simulink model "Milford"  (R2017a)
settings: Solver=FixedStepAuto  StartTime=0.0  StopTime=Cycle_End  FixedStep=0.01  MaxStep=0.01  RelTol=1e-3  EnableMultiTasking=on
PostLoadFcn:
  | , if any(exist('dsrtsu_mdlpostloadfcn', 'file') == [2, 3, 6]), try dsrtsu_mdlpostloadfcn('Execute', bdroot); catch fprintf('Error in PostLoadFcn (dsrtsu_mdlpostloadfcn) for model "%s":\n %s\n', bdroot, lasterr); end, end,
undefined symbols (not defined in the file): Actuators, APP1_OOR, APP2_OOR, APP_Mismatch, Brk_Flt, cal, ClutchEngag, DiscIntNeverNeededParam, eng, Engine, EngOverTemp, ENGTRQ_MSMCH_Degraded_CP, ENGTRQ_MSMCH_ErrCritical_CP, ENGTRQ_MSMCH_LimpHome_CP, EngTrqMismatch, ESSOverTemp, gb, Gearbox, KeyPos_Flt, lib_Actuators, lib_Sensors_2017a, lib_Transmission, Loss, LossCAN, MCUOverTemp, mot, MotDirMismatch, MotOverTemp, MotTrqMismatch, mph2kph, PRNDL_Flt, Ratio, RegenFault, Sensors, Spd, time, Transmission
libraries: simulink x110, powerlib_meascontrol x6, EC2_libraries x5, dspsigops x3, lib_Chassis x1, lib_DCDC x1, lib_Differential x1, lib_HVESS x1, lib_Engine x1, lib_OBC x1, Transmission_Validation x1, lib_Wheels x1
(part 9 of 9)

== stateflow chart Milford/Controller_with_Transmission_Manager1/HSC/Powertrain Manager/HV Manager/BMS_Manager/ESS_Manager ==
  state Fault_light_OFF
    entry: GFD_Light=0;
  state Ground_Fault
    entry:
    HV_State=-7;
    GFD_Light=1
  state Voltage_Fault
  state HVIL_Fault
    entry: MO_BMS_Sollmodus=0;
    HV_State=-8
  state HV_Startup
    state Drive_State
      entry:  HV_State=1;
      T_15=1;
      T_30=1;
      HVDischarge=0;
    state Contactor
      entry:
      T_30C=1;
    state Clear_Faults
      entry:
      Diag_Rq_Fktnl_Data_OBD_byte_0 =1;
      Diag_Rq_Fktnl_Data_OBD_byte_1=4;
      Diag_Rq_Fktnl_Data_OBD_byte_2=0;
      Diag_Rq_Fktnl_Data_OBD_byte_3=0;
      Diag_Rq_Fktnl_Data_OBD_byte_4=0;
      Diag_Rq_Fktnl_Data_OBD_byte_5=0;
      Diag_Rq_Fktnl_Data_OBD_byte_6=0;
      Diag_Rq_Fktnl_Data_OBD_byte_7=0;
      HV_State=2;
    state Charge_Wake
      entry: chga_wake=1;
      HV_State=3;
    state Drive_Wake
      entry: veh_wake=1;
      HV_State=8;
    state BMS_Enable_Charge
      entry: MO_BMS_Sollmodus=0;
      % T_15=1;
      % T_30C=1;
      HV_State=4;
    state BMS_Enable_Drive
      entry: MO_BMS_Sollmodus=0;
      HV_State=9;
    state Power_Contactors_Drive
      en: MO_BMS_Sollmodus=0;
      HV_State=10;
    state Power_Contactors_Charge
      en: MO_BMS_Sollmodus=0;
      %T_30C=1;
      HV_State=5;
    state Close_Contactors_Drive
      entry:
      MO_BMS_Sollmodus=1;
      HV_State=11;
    state Close_Contactors_Charge
      entry:
      MO_BMS_Sollmodus=1;
      HV_State=6;
    state Time_delay
    state Ready_to_Charge
      entry: ReadyToCharge=1;
      ISO_Hybrid_01_Req = 1;
      HV_State=7;
    state Ready_to_Drive
      entry: ReadyToDrive=1;
      ISO_Hybrid_01_Req = 1;
      HV_State=12;
    (default) -> Contactor
    Contactor -> Drive_State : after(0.25,sec)
    Drive_State -> Clear_Faults : after(0.1,sec)
    Clear_Faults -> Charge_Wake [order 1] : [plugged]
    Clear_Faults -> Drive_Wake [order 2] : %after(0.1,sec)
    Drive_Wake -> BMS_Enable_Drive : [BMS_Fehler_Pilot==0 ]
    Charge_Wake -> BMS_Enable_Charge : [BMS_Fehler_Pilot==0 ]
    BMS_Enable_Charge -> Power_Contactors_Charge : [BMS_Init_abgeschlossen]
    BMS_Enable_Drive -> Power_Contactors_Drive : [BMS_Init_abgeschlossen]
    Power_Contactors_Drive -> Close_Contactors_Drive : [closeMaincReq]
    Power_Contactors_Charge -> Close_Contactors_Charge : [closeMaincReq]
    Close_Contactors_Charge -> Time_delay : [BMS_Fehler_HS_offen==0&&(BMS_IstModus==4||BMS_IstModus==1)]
    Close_Contactors_Drive -> Ready_to_Drive : [BMS_Fehler_HS_offen==0&&BMS_IstModus==1]
    Time_delay -> Ready_to_Charge : after(1,sec)
    Ready_to_Drive -> Ready_to_Charge : [plugged]
    Ready_to_Charge -> Ready_to_Drive : [plugged==0]
  note: // Rev 2_14_2017
      | Added plugged to Off-On transition
      | Added EnableInverter to charge path
      | Changed IstModus to 1 at the end of charge path
      |
      | Create HV On Request block to request charging when vehicle is off
  state HV_Shudown
    state Open_Contactors
      entry: MO_BMS_Sollmodus=0;
      HV_State=-1;
      ISO_Hybrid_01_Req = 0;
    state ShutDown_T30C
      entry: T_30C=0;
    state Discharge_Bus
      entry: HVDischarge=1;
      HV_State=-2;
    state Disable_BCM_1
      entry: T_15=0;
      HVDischarge=0;
      HV_State=-3;
    state Disable_BCM_2
      entry: T_30=0;
      HVDischarge=0;
      HV_State=-4;
    state Send_BCM_to_Sleep
      en: MO_SleepAckn =1;
      T_15=0;
      T_30=0;
      HV_State=-5;
    state Shutdown_Complete
      entry: Shutdown_Complete=1;
      HV_State=-6;
    (default) -> Open_Contactors
    Open_Contactors -> ShutDown_T30C : after(2,sec)
    ShutDown_T30C -> Discharge_Bus : [BMS_IstModus==5]
    Discharge_Bus -> Disable_BCM_1 : [BMS_Spannung_ZwKr<30]
    Disable_BCM_1 -> Disable_BCM_2 : [BMS_IstStrom<0.02]
    Disable_BCM_2 -> Send_BCM_to_Sleep
    Send_BCM_to_Sleep -> Shutdown_Complete : [BMS_SleepInd]
  note: //Rev 8_21_2017
      | //Removed all engine related conditions
      | //Removed EngRunATV
  Voltage_Fault -> HV_Shudown [order 1] : after(0.5, sec)
  Ground_Fault -> Fault_light_OFF : [(ISOfault==0&&KeyPos==1)||(ISOfault==0&&KeyPos==0&&plugged==1)]
  HV_Shudown -> Ground_Fault [order 2] : [ISOfault==1]
  Fault_light_OFF -> HV_Shudown
  HV_Startup -> Ground_Fault [order 3] : [ISOfault==1]
  HV_Startup -> HVIL_Fault [order 4] : [BMS_Fehler_Pilot]
  HVIL_Fault -> HV_Shudown : [BMS_Fehler_Pilot==0]
  HV_Startup -> Voltage_Fault [order 2] : after(5,sec)
      | [BMS_Spannung_ZwKr<50&&EngRunAtv]
  Voltage_Fault -> HV_Startup [order 2] : after(1,sec)
  (default) -> HV_Shudown
  HV_Shudown -> HV_Startup [order 1] : [HV_req==1||plugged||EngRunAtv]
  HV_Startup -> HV_Shudown [order 1] : [closeMaincReq==0&&plugged==0]
      | {ReadyToDrive = 0;
      | ReadyToCharge = 0;}
  data: data local; ISOfault input; plugged input; BMS_Fehler_HS_offen input; BMS_Fehler_Pilot input; BMS_Init_abgeschlossen input; BMS_IstModus input; BMS_IstSpannung input; BMS_IstStrom input; BMS_SleepInd input; Diag_Rq_Fktnl_Data_OBD_byte_0 output; Diag_Rq_Fktnl_Data_OBD_byte_1 output; Diag_Rq_Fktnl_Data_OBD_byte_2 output; Diag_Rq_Fktnl_Data_OBD_byte_3 output; Diag_Rq_Fktnl_Data_OBD_byte_4 output; Diag_Rq_Fktnl_Data_OBD_byte_5 output; Diag_Rq_Fktnl_Data_OBD_byte_6 output; Diag_Rq_Fktnl_Data_OBD_byte_7 output; ISO_Hybrid_01_Req output; MO_SleepAckn output; MO_BMS_Sollmodus output; T_15 output; T_30 output; T_30C output; veh_wake output; chga_wake output; HVDischarge output; HV_State output; ReadyToDrive output; ReadyToCharge output; Shutdown_Complete output; HV_req input boolean; BMS_Spannung_ZwKr input; NMH_BMS_Car_WakeUp input; NMH_Normal_Mode_1 input; NMH_BMS_Normal_Mode_2 input; NMH_BMS_Start_1 input; NMH_BMS_Start_2 input; timer local; KeyPos input; GFD_Light output; EngRunAtv input; closeMaincReq input boolean

== stateflow chart Milford/Controller_with_Transmission_Manager1/HSC/Powertrain Manager/HV Manager/DCDC Manager/DCDCManager ==
  state DCDC_Initialization
    state Initialization
      entry: DCDC_State = 1;
    state Power_On
      entry: DCmode = 1;
      DCDC_State = 2;
      VoltageHV = 0;
      VoltageLV =14;
      CurrentHV = 20;
      CurrentLV = 173;
    (default) -> Initialization
    Initialization -> Power_On : [ContactorsFailed == 0]
  state Delay
  state DCDC_Off
    entry: DCDC_State = 4;
    DCmode = 0;
  (default) -> DCDC_Initialization
  Delay -> DCDC_Initialization : after(5,sec)
  DCDC_Initialization -> DCDC_Off : [INV_state == 14 || ...
      | ContactorsFailed == 1|| ...
      | mode == 7]
  DCDC_Off -> Delay : [(INV_state == 3 || INV_state == 8) && ...
      | ContactorsFailed == 0&&...
      |  (powerMode ==1|| powerMode == 2 || powerMode == 3)]
  data: ContactorsFailed input; DCmode output; VoltageHV output; CurrentHV output; VoltageLV output; CurrentLV output; INV_state input; DCDC_State output; mode input; powerMode input

== stateflow chart Milford/Controller_with_Transmission_Manager1/HSC/Powertrain Manager/HV Manager/Inverter Manager/MCU_Manager  ==
  state MCU_Initialization
    state MCU_Request_Standby
      en:
      MCU_State = 1;
      RequestedStateINV = 3;
      CAN_Activation = 1;
    state Power_Off_INVCON
      entry:
      MCU_State = 0;
      INVCON_Power =0;
    state Power_On_INVCON
      en:MCU_State = 2;
      INVCON_Power =1;
    state HV_CAN_Actuation_Fault
      en:
      MCU_State = -1;
      CAN_Activation = 0;
    state INVCON_Power_Fault
      en:
      MCU_State = -2;
      INVCON_Power =0;
      CAN_Activation = 0;
    Power_Off_INVCON -> (junction 18) : {Timer=0;}
    (junction 18) -> MCU_Request_Standby [order 1] : [HVCAN_State]
    (default) -> Power_Off_INVCON
    HV_CAN_Actuation_Fault -> (junction 18) : [HVCAN_State]
    (junction 18) -> HV_CAN_Actuation_Fault [order 2] : after(3,sec)
    INVCON_Power_Fault -> (junction 18) : [~INVCON_Power_Feedback]
    MCU_Request_Standby -> Power_On_INVCON : after(5,sec)
    Power_On_INVCON -> INVCON_Power_Fault : after(5,sec)
        | [INV_State ~= 3]
  state MCU_ChargeMode
    state MCU_Ready
      en:
      MCU_State = 7;
    state MCU_Off
      en:
      MCU_State = 8;
      RequestedStateINV = 3;
    (default) -> MCU_ChargeMode.MCU_Ready
    MCU_ChargeMode.MCU_Ready -> MCU_ChargeMode.MCU_Off : [~ReadyToCharge]
  state MCU_TorqueMode
    state MCU_Enable
      en:MCU_State = 4;
      RequestedStateINV = 8;
      during: Timer = Timer + 1;
    state MCU_Ready
      en:
      MCU_State = 3;
    state MCU_Running
      en:
      MCU_State =5;
    state TorqueCommand_Reject_Fault
      en:
      MCU_State = -3;
    state MCU_Stop
      en:
      MCU_State = 6;
      RequestedStateINV = 3;
    (default) -> MCU_TorqueMode.MCU_Ready
    MCU_Enable -> (junction 35)
    (junction 35) -> MCU_Running [order 1] : [INV_State == 8]
    MCU_TorqueMode.MCU_Ready -> MCU_Enable : [EnableInverter]
        | {Timer = 0;}
    (junction 35) -> TorqueCommand_Reject_Fault [order 2] : after(5,sec)
    MCU_Running -> MCU_Stop : [~ReadyToDrive]
  state MCU_Shutdown
    state MCU_Off
      en:
      MCU_State = 10;
      RequestedStateINV = 0;
      during: Timer=Timer+1;
    state MCU_RdyForShtDwn
      en:
      MCU_State = 9;
    state MCU_Shtdwn_Cmplt
      en:
      MCU_State = 11;
      INVCON_Power =0;
      CAN_Activation = 0;
    state Motor_Isolate
      en:
      MCU_State = -5;
      INVCON_Power = 0;
      Motor_Torque_Command = 0;
    state ShutdownReq_Reject_Fault
      en:
      MCU_State = -4;
    (default) -> MCU_RdyForShtDwn
    MCU_RdyForShtDwn -> MCU_Shutdown.MCU_Off : [~EnableInverter]
        | {Timer = 0;}
    MCU_Shutdown.MCU_Off -> (junction 55)
    (junction 55) -> MCU_Shtdwn_Cmplt [order 2] : [INV_State == 0]
    (junction 55) -> ShutdownReq_Reject_Fault [order 1] : after(5,sec)
        | [INV_State == 14]
    ShutdownReq_Reject_Fault -> Motor_Isolate : after(3,sec)
  (default) -> MCU_Initialization
  MCU_Shutdown -> MCU_Initialization : [EnableInverter]
  MCU_TorqueMode -> MCU_Initialization [order 1] : [INV_State == 14]
  MCU_Initialization -> MCU_TorqueMode [order 2] : [INV_State == 3 &&...
      |  INVCON_Power_Feedback && ReadyToDrive]
  MCU_Initialization -> MCU_ChargeMode [order 1] : [INV_State == 3 &&...
      |  INVCON_Power_Feedback && ReadyToCharge]
  MCU_ChargeMode -> MCU_Initialization [order 2] : [INV_State == 14]
  MCU_TorqueMode -> MCU_Shutdown [order 2] : [INV_State == 3 && ~ReadyToDrive]
  MCU_ChargeMode -> MCU_Shutdown [order 1] : [INV_State == 3 && ~ReadyToCharge]
  data: ReadyToDrive input boolean; ReadyToCharge input; HVCAN_State input boolean; INVCON_Power_Feedback input; INV_State input; INV_CurrentHV input; Timer local double; MCU_State output; EnableInverter input boolean; ShutdownCurrent input; Motor_Torque_Command output; INVCON_Power output double; RequestedStateINV output; CAN_Activation output

== stateflow chart Milford/Controller_with_Transmission_Manager1/HSC/Powertrain Manager/Torque Distribution/Sport Mode Enable/Sports Mode Logic ==
  state Sport_Mode
    entry:
    Driver_Mode=2;
  state Hybrid_Mode
    entry:
    Driver_Mode=1;
  Hybrid_Mode -> Sport_Mode : [Voltage_Input>3.5&&Voltage_Input<3.9]
  (default) -> Hybrid_Mode
  Sport_Mode -> Hybrid_Mode : [Voltage_Input>1.8&&Voltage_Input<2.2]
  data: Voltage_Input input; Driver_Mode output

== stateflow chart Milford/Controller_with_Transmission_Manager1/HSC/Powertrain Manager/Torque Distribution/Supervisory  Control  Logic1 ==
  note: 
  state VehOn
    en:
    mode = 6;
    powerMode = 1;
    HV_Req=1;
    ClutchEngage = 2000;
  note: Tranmission Shift Level Position (ShftLvrPos):
  state VehOffOrAcc
    en:
    mode=0;
    powerMode = 0;
    EnablePrplsn = 0;
    HV_Req=0;
    closeMaincReq=0;
    ClutchEngage = 2000;
  state Close_Contactors
    en:
    closeMaincReq=1;
    ClutchEngage = 2000;
  state VehShutdown
    en:
    powerMode = 1;
    EnablePrplsn = 0;
    EngOnReq = 0;
    MotTrqReq = 0;
    EngAppReq = 0;
    EnableInverter=0;
    mode=8;
    ClutchEngage = 2000;
    closeMaincReq=0;
    HV_Req=0;
  state Charging
    en:
    mode = 9;
    powerMode = 3;
    HV_Req=1;
    closeMaincReq = 1;
    EnablePrplsn = 0;
    EnableInverter = 0;
  state EnablePropulsion
    en:
    mode=7;
    EnablePrplsn = 1;
    ClutchEngage = 2000;
  note: System Power Mode (KeyPos):
  state VehReady
    en:
    powerMode = 2;
    state Eng_Only_Mode
      en:
      EngOnReq = 1;
      mode=3;
      du:
      MotTrqReq = 0;
      closeMaincReq=0;
      EngTrq = EngTrqCalc(drvAPP,EngSpd,ShftLvrPos,DrvIntdAxleTrq,TransRatio);
      EngAppReq=drvAPP;
      state T = EngTrqCalc(APP,EngSpeed,Shifter,DrvIntdAxleTrq,TransRatio) [function]
      state APP = EngTrq2EngApp(T,TransRatio) [function]
    state Clutch_Engage1
      en:
      MotTrqReq = 0;
      EngAppReq = 0;
      state EngStart1
        en: EngOnReq = 1;
      state EngApp = SyncCtrl(EngSpeed,MotorSpeed) [function]
      state EngageClutch
        en:
        ClutchEngage = 0;
      state EngSpdSync
        du:
        EngAppReq = SyncCtrl(EngSpd,MotSpd);
      state EngageClutch1
        en:
        ClutchEngage = 0;
      (default) -> (junction 1687)
      (junction 1687) -> VehReady.Clutch_Engage1.EngStart1 [order 2] : [ClutchEngage == 2000]
      (junction 1687) -> VehReady.Clutch_Engage1.EngageClutch [order 1] : [ClutchEngage == 0]
      VehReady.Clutch_Engage1.EngStart1 -> VehReady.Clutch_Engage1.EngSpdSync : [EngRunAtv]
      VehReady.Clutch_Engage1.EngSpdSync -> VehReady.Clutch_Engage1.EngageClutch1
    state CD_Mode
      en:
      mode=1;
      state Drive_mode
        en:
        mode=11;
        Brkmode=0;
        EngOnReq=0;
        du:
        MotTrqReq = MotTrqCalc2(drvAPP,ShftLvrPos,DrvIntdAxleTrq,TransRatio);
        EngAppReq=0;
        ClutchEngage=2000;
        state MotTrq = MotTrqCalc2(APP,ShftLvrPos,DrvIntdAxleTrq,TransRatio) [function]
      state Brake_mode
        en:
        mode=12;
        EngAppReq=0;
        state Regen_mode
          en:
          Brkmode=1;
          du:
          MotTrqReq=MotTrqCalc1(BrkPdlPos,VehicleSpeed,...
          ShftLvrPos,MotSpd,TransRatio,IntdAxleTrq);
        state No_regen
          en:
          Brkmode=2;
          du:
          MotTrqReq=MotTrqCalc2(ShftLvrPos,TransRatio);
        state Temp_delay
        state Temp_delay1
        state T = MotTrqCalc1(BPP,VehSpd,ShftLvrPos,MotSpeed,TransRatio,IntdAxleTrq) [function]
        state T = MotTrqCalc2(ShftLvrPos,TransRatio) [function]
        (default) -> VehReady.CD_Mode.Brake_mode.No_regen
        VehReady.CD_Mode.Brake_mode.Regen_mode -> VehReady.CD_Mode.Brake_mode.Temp_delay : [RegenBrkDisable||SoC>=80||ABSAtv||Regen_fault]
        VehReady.CD_Mode.Brake_mode.Temp_delay -> VehReady.CD_Mode.Brake_mode.No_regen : after(0.25,sec)
        VehReady.CD_Mode.Brake_mode.Temp_delay1 -> VehReady.CD_Mode.Brake_mode.Regen_mode : after(0.25,sec)
        VehReady.CD_Mode.Brake_mode.No_regen -> VehReady.CD_Mode.Brake_mode.Temp_delay1 : [RegenBrkDisable == 0&&SoC<80&&ABSAtv==0&&Regen_fault==0]
      state Time_delay
      state Time_delay1
      (default) -> VehReady.CD_Mode.Drive_mode
      VehReady.CD_Mode.Drive_mode -> VehReady.CD_Mode.Time_delay : [BrkPdlPos>0&&IntdAxleTrq<0]
      VehReady.CD_Mode.Time_delay -> VehReady.CD_Mode.Brake_mode : after(0.25,sec)
      VehReady.CD_Mode.Time_delay1 -> VehReady.CD_Mode.Drive_mode : after(0.25,sec)
      VehReady.CD_Mode.Brake_mode -> VehReady.CD_Mode.Time_delay1 : [drvAPP>0&&IntdAxleTrq>=0]
    state Sport_Mode
      en:
      mode=4;
      EngOnReq = 1;
      state Brake_mode
        du:
        EngTrq =0;
        EngAppReq = 0;
        state regen_mode
          en:
          Brkmode=1;
          du:
          MotTrqReq=MotTrqCalc1(BrkPdlPos,VehicleSpeed,...
          ShftLvrPos,MotSpd,IntdAxleTrq,TransRatio);
        state No_regen
          en:
          Brkmode=2;
          du:
          MotTrqReq=0;
        state Temp_delay
        state Temp_delay1
        state T = MotTrqCalc1(BPP,VehSpd,ShftLvrPos,MotSpeed,IntdAxleTrq,TransRatio) [function]
        (default) -> VehReady.Sport_Mode.Brake_mode.No_regen
        VehReady.Sport_Mode.Brake_mode.regen_mode -> VehReady.Sport_Mode.Brake_mode.Temp_delay : [RegenBrkDisable||SoC>=80||ABSAtv||Regen_fault]
        VehReady.Sport_Mode.Brake_mode.Temp_delay -> VehReady.Sport_Mode.Brake_mode.No_regen : after(0.5,sec)
        VehReady.Sport_Mode.Brake_mode.No_regen -> VehReady.Sport_Mode.Brake_mode.Temp_delay1 : [!RegenBrkDisable&&SoC<80&&ABSAtv==0&&!Regen_fault]
        VehReady.Sport_Mode.Brake_mode.Temp_delay1 -> VehReady.Sport_Mode.Brake_mode.regen_mode : after(1,sec)
      state Drive_mode
        du:
        MotTrqReq = MotTrqCalc(drvAPP,ShftLvrPos,MotSpd,DrvIntdAxleTrq,TransRatio);
        EngTrq = EngTrqCalc(drvAPP,EngSpd,ShftLvrPos,DrvIntdAxleTrq,TransRatio);
        EngAppReq = EngTrq2EngApp(EngTrq,TransRatio);
      state Time_delay
      state Time_delay1
      state T = MotTrqCalc(APP,Shifter,MotSpeed,DrvIntdAxleTrq,TransRatio) [function]
      state T = EngTrqCalc(APP,EngSpeed,Shifter,DrvIntdAxleTrq,TransRatio) [function]
      state APP = EngTrq2EngApp(Trq,TransRatio) [function]
      (default) -> VehReady.Sport_Mode.Drive_mode
      VehReady.Sport_Mode.Drive_mode -> VehReady.Sport_Mode.Time_delay : [BrkPdlPos>0&&IntdAxleTrq<0]
      VehReady.Sport_Mode.Time_delay -> VehReady.Sport_Mode.Brake_mode
      VehReady.Sport_Mode.Time_delay1 -> VehReady.Sport_Mode.Drive_mode
      VehReady.Sport_Mode.Brake_mode -> VehReady.Sport_Mode.Time_delay1 : [drvAPP>0&&IntdAxleTrq>=0]
    state Clutch_Engage3
      en:
      MotTrqReq = 0;
      EngAppReq = 0;
      ClutchEngage = 0;
      state EngApp = SyncCtrl(EngSpeed,MotorSpeed) [function]
      state EngStart
        en: EngOnReq = 1;
      (default) -> VehReady.Clutch_Engage3.EngStart : [VehicleSpeed < 1 && TransEstGear == 15]
    state Clutch_Engage
      en:
      MotTrqReq = 0;
      EngAppReq = 0;
      state EngStart1
        en: EngOnReq = 1;
      state EngApp = SyncCtrl(EngSpeed,MotorSpeed) [function]
      state EngageClutch
        en:
        ClutchEngage = 0;
      state EngSpdSync
        du:
        EngAppReq = SyncCtrl(EngSpd,MotSpd);
      state EngStart
        en: EngOnReq = 1;
      state EngageClutch1
        en:
        ClutchEngage = 0;
      (default) -> (junction 1792)
      (junction 1792) -> VehReady.Clutch_Engage.EngStart1 [order 2] : [VehicleSpeed >= 1]
      (junction 1792) -> VehReady.Clutch_Engage.EngageClutch [order 1] : [VehicleSpeed < 1]
      VehReady.Clutch_Engage.EngStart1 -> VehReady.Clutch_Engage.EngSpdSync : [EngRunAtv]
      VehReady.Clutch_Engage.EngageClutch -> VehReady.Clutch_Engage.EngStart : [ClutchEngage == 0]
      VehReady.Clutch_Engage.EngSpdSync -> VehReady.Clutch_Engage.EngageClutch1 : [abs(EngSpd - MotSpd) < 100]
    state CS_Mode
      state Engine_Charge
        en:
        mode=2;
        state Drive_Mode
          en:
          mode=20;
          Brkmode=0;
          du:
          EngTrq = EngTrqCalc(EngSpd,drvAPP,VehicleSpeed,ShftLvrPos,DrvIntdAxleTrq,TransRatio,SoC);
          EngAppReq = EngTrq2EngApp(EngTrq,TransRatio);
          MotTrqReq = MotTrqCalc2(drvAPP,ShftLvrPos,DrvIntdAxleTrq,TransRatio,SoC,SW_CS_ON,Faked_SoC,EngTrq,MotSpd);
          state APP = EngTrq2EngApp(Trq,TransRatio) [function]
          state Trq = EngTrqCalc(EngSpeed,APP,VehSpd,ShftLvrPos,DrvIntdAxleTrq,TransRatio,SOC) [function]
          state MotTrq = MotTrqCalc2(APP,ShftLvrPos,DrvIntdAxleTrq,TransRatio,SoC,CS_On,Faked_SoC,MotSpd,Trq) [function]
        state Brake_mode1
          en:
          mode=21;
          EngAppReq=0.51;
          state regen_mode
            en:
            Brkmode=1;
            du:
            MotTrqReq=MotTrqCalc1(BrkPdlPos,VehicleSpeed,...
            ShftLvrPos,MotSpd,TransRatio,IntdAxleTrq);
          state No_regen
            en:
            Brkmode=2;
            du:
            MotTrqReq=MotTrqCalc2(ShftLvrPos,TransRatio);
          state Temp_delay
          state Temp_delay1
          state T = MotTrqCalc1(BPP,VehSpd,ShftLvrPos,MotSpeed,TransRatio,IntdAxleTrq) [function]
          state T = MotTrqCalc2(ShftLvrPos,TransRatio) [function]
          (default) -> VehReady.CS_Mode.Engine_Charge.Brake_mode1.No_regen
          VehReady.CS_Mode.Engine_Charge.Brake_mode1.regen_mode -> VehReady.CS_Mode.Engine_Charge.Brake_mode1.Temp_delay : [RegenBrkDisable||SoC>=80||ABSAtv||Regen_fault]
          VehReady.CS_Mode.Engine_Charge.Brake_mode1.Temp_delay -> VehReady.CS_Mode.Engine_Charge.Brake_mode1.No_regen : after(0.25,sec)
          VehReady.CS_Mode.Engine_Charge.Brake_mode1.Temp_delay1 -> VehReady.CS_Mode.Engine_Charge.Brake_mode1.regen_mode : after(0.25,sec)
          VehReady.CS_Mode.Engine_Charge.Brake_mode1.No_regen -> VehReady.CS_Mode.Engine_Charge.Brake_mode1.Temp_delay1 : [RegenBrkDisable == 0&&EngSpd>1000&&SoC<80&&ABSAtv==0&&Regen_fault==0]
        state Time_delay3
        state Time_delay2
        (default) -> Drive_Mode
        Drive_Mode -> Time_delay3 : [BrkPdlPos>0 && IntdAxleTrq<0]
        Time_delay3 -> Brake_mode1 : after(0.25,sec)
        Time_delay2 -> Drive_Mode : after(0.25,sec)
        Brake_mode1 -> Time_delay2 : [drvAPP>0&&IntdAxleTrq>=0]
      state Motor_Assist
        en:
        mode=3;
        state Drive_mode
          en:
          mode=30;
          Brkmode=0;
          du:
          EngTrq = 0;
          EngAppReq = 0;
          MotTrqReq = MotTrqCalc2(drvAPP,DrvIntdAxleTrq,TransRatio,ShftLvrPos);
          state MotTrq = MotTrqCalc2(APP,DrvIntdAxleTrq,TransRatio,ShftLvrPos) [function]
        state Brake_mode
          en:
          mode=31;
          EngAppReq=0.51;
          state Regen_mode
            en:
            Brkmode=1;
            du:
            MotTrqReq=MotTrqCalc1(BrkPdlPos,VehicleSpeed,...
            ShftLvrPos,MotSpd,TransRatio,IntdAxleTrq);
          state No_regen
            en:
            Brkmode=2;
            du:
            MotTrqReq=MotTrqCalc2(ShftLvrPos,TransRatio);
          state Temp_delay
          state Temp_delay1
          state T = MotTrqCalc1(BPP,VehSpd,ShftLvrPos,MotSpeed,TransRatio,IntdAxleTrq) [function]
          state T = MotTrqCalc2(ShftLvrPos,TransRatio) [function]
          (default) -> VehReady.CS_Mode.Motor_Assist.Brake_mode.No_regen
          VehReady.CS_Mode.Motor_Assist.Brake_mode.Regen_mode -> VehReady.CS_Mode.Motor_Assist.Brake_mode.Temp_delay : [RegenBrkDisable||SoC>=80||ABSAtv||Regen_fault]
          VehReady.CS_Mode.Motor_Assist.Brake_mode.Temp_delay -> VehReady.CS_Mode.Motor_Assist.Brake_mode.No_regen : after(0.25,sec)
          VehReady.CS_Mode.Motor_Assist.Brake_mode.Temp_delay1 -> VehReady.CS_Mode.Motor_Assist.Brake_mode.Regen_mode : after(0.25,sec)
          VehReady.CS_Mode.Motor_Assist.Brake_mode.No_regen -> VehReady.CS_Mode.Motor_Assist.Brake_mode.Temp_delay1 : [RegenBrkDisable == 0&&EngSpd>1000&&SoC<80&&ABSAtv==0&&Regen_fault==0]
        state Time_delay
        state Time_delay1
        (default) -> VehReady.CS_Mode.Motor_Assist.Drive_mode
        VehReady.CS_Mode.Motor_Assist.Drive_mode -> VehReady.CS_Mode.Motor_Assist.Time_delay : [BrkPdlPos>0&&IntdAxleTrq<0]
        VehReady.CS_Mode.Motor_Assist.Time_delay -> VehReady.CS_Mode.Motor_Assist.Brake_mode : after(0.25,sec)
        VehReady.CS_Mode.Motor_Assist.Time_delay1 -> VehReady.CS_Mode.Motor_Assist.Drive_mode : after(0.25,sec)
        VehReady.CS_Mode.Motor_Assist.Brake_mode -> VehReady.CS_Mode.Motor_Assist.Time_delay1 : [drvAPP>0&&IntdAxleTrq>=0]
      state Time_Delay
      state Time_Delay1
      state Clutch_Engage
        en:
        MotTrqReq = 0;
        EngAppReq = 0;
        state EngApp = SyncCtrl(EngSpeed,MotorSpeed) [function]
        state EngStart1
          en: EngOnReq = 1;
        state EngSpdSync
          du:
          EngAppReq = SyncCtrl(EngSpd,MotSpd);
        state EngageClutch1
          en:
          ClutchEngage = 0;
        (default) -> VehReady.CS_Mode.Clutch_Engage.EngStart1
        VehReady.CS_Mode.Clutch_Engage.EngStart1 -> VehReady.CS_Mode.Clutch_Engage.EngSpdSync : [EngRunAtv]
        VehReady.CS_Mode.Clutch_Engage.EngSpdSync -> VehReady.CS_Mode.Clutch_Engage.EngageClutch1 : [abs(EngSpd - MotSpd) < 100]
      state Motor_Assist1 [commented out]
        en:
        mode=3;
        state Drive_mode [commented out]
          en:
          mode=30;
          Brkmode=0;
          du:
          EngTrq = EngTrqCalc(EngSpd,drvAPP,VehicleSpeed,ShftLvrPos,DrvIntdAxleTrq,TransRatio);
          EngAppReq = EngTrq2EngApp(EngTrq,TransRatio);
          MotTrqReq = MotTrqCalc2(drvAPP,EngFdbkTrq,ShftLvrPos,DrvIntdAxleTrq,TransRatio,EngTrq);
          state APP = EngTrq2EngApp(Trq,TransRatio) [function] [commented out]
          state MotTrq = MotTrqCalc2(APP,EngFdbkTrq,ShftLvrPos,DrvIntdAxleTrq,TransRatio,Trq) [function] [commented out]
          state Trq = EngTrqCalc(EngSpeed,APP,VehSpd,ShftLvrPos,DrvIntdAxleTrq,TransRatio) [function] [commented out]
        state Brake_mode [commented out]
          en:
          mode=31;
          EngAppReq=0.51;
          state Regen_mode [commented out]
            en:
            Brkmode=1;
            du:
            MotTrqReq=MotTrqCalc1(BrkPdlPos,VehicleSpeed,...
            ShftLvrPos,MotSpd,TransRatio,IntdAxleTrq);
          state No_regen [commented out]
            en:
            Brkmode=2;
            du:
            MotTrqReq=MotTrqCalc2(ShftLvrPos,TransRatio);
          state Temp_delay [commented out]
          state Temp_delay1 [commented out]
          state T = MotTrqCalc1(BPP,VehSpd,ShftLvrPos,MotSpeed,TransRatio,IntdAxleTrq) [function] [commented out]
          state T = MotTrqCalc2(ShftLvrPos,TransRatio) [function] [commented out]
          (default) -> VehReady.CS_Mode.Motor_Assist1.Brake_mode.No_regen [commented out]
          VehReady.CS_Mode.Motor_Assist1.Brake_mode.Regen_mode -> VehReady.CS_Mode.Motor_Assist1.Brake_mode.Temp_delay [commented out] : [RegenBrkDisable||SoC>=80||ABSAtv||Regen_fault]
          VehReady.CS_Mode.Motor_Assist1.Brake_mode.Temp_delay -> VehReady.CS_Mode.Motor_Assist1.Brake_mode.No_regen [commented out] : after(0.25,sec)
          VehReady.CS_Mode.Motor_Assist1.Brake_mode.Temp_delay1 -> VehReady.CS_Mode.Motor_Assist1.Brake_mode.Regen_mode [commented out] : after(0.25,sec)
          VehReady.CS_Mode.Motor_Assist1.Brake_mode.No_regen -> VehReady.CS_Mode.Motor_Assist1.Brake_mode.Temp_delay1 [commented out] : [RegenBrkDisable == 0&&EngSpd>1000&&SoC<80&&ABSAtv==0&&Regen_fault==0]
        state Time_delay [commented out]
        state Time_delay1 [commented out]
        (default) -> VehReady.CS_Mode.Motor_Assist1.Drive_mode [commented out]
        VehReady.CS_Mode.Motor_Assist1.Drive_mode -> VehReady.CS_Mode.Motor_Assist1.Time_delay [commented out] : [BrkPdlPos>0&&IntdAxleTrq<0]
        VehReady.CS_Mode.Motor_Assist1.Time_delay -> VehReady.CS_Mode.Motor_Assist1.Brake_mode [commented out] : after(0.25,sec)
        VehReady.CS_Mode.Motor_Assist1.Time_delay1 -> VehReady.CS_Mode.Motor_Assist1.Drive_mode [commented out] : after(0.25,sec)
        VehReady.CS_Mode.Motor_Assist1.Brake_mode -> VehReady.CS_Mode.Motor_Assist1.Time_delay1 [commented out] : [drvAPP>0&&IntdAxleTrq>=0]
      (default) -> Engine_Charge
      Engine_Charge -> Time_Delay : [(SW_CS_ON==0&&SoC > CS_SOC_MAX) || (SW_CS_ON==0&&VehicleSpeed >40 &&...
          |  SoC > (CS_SOC_MIN+5))||(SW_CS_ON&&SoC>(Faked_SoC+5))]
      Time_Delay -> Motor_Assist : after(1,sec)
      Time_Delay1 -> Engine_Charge : after(1,sec)
      Motor_Assist -> VehReady.CS_Mode.Clutch_Engage : [SoC < CS_SOC_MIN&& BrkPdlPos == 0||...
          | (SW_CS_ON&&SoC<Faked_SoC)]
      VehReady.CS_Mode.Clutch_Engage -> Time_Delay1 : [ClutchEngage==1]
    (default) -> Eng_Only_Mode : [eSystemStatus==0&&...
        | iceSystemStatus>1]
    CD_Mode -> Clutch_Engage1 [order 2] : [(SoC < 0.05 && ...
        | iceSystemStatus == 2)||...
        | (iceSystemStatus==2&&eSystemStatus == 0)]
    Clutch_Engage1 -> Eng_Only_Mode : after(1,sec)
        | [ClutchEngage==0&&...
        | EngRunAtv == 1]
    CD_Mode -> Clutch_Engage3 [order 3] : [SportModeEnabled == 1&&...
        | iceSystemStatus>1&&eSystemStatus>1]
    Clutch_Engage3 -> Sport_Mode : [EngRunAtv]
    Eng_Only_Mode -> CD_Mode [order 2] : [(SoC > CD_SOC_MIN && ...
        | eSystemStatus == 2) || ...
        | (iceSystemStatus == 0&&eSystemStatus)]
    Sport_Mode -> CD_Mode [order 1] : [SportModeEnabled == 0&&iceSystemStatus&&eSystemStatus]
    Eng_Only_Mode -> CS_Mode [order 1] : [SoC<CS_SOC_MIN&&SoC>0.1]
    CS_Mode -> Eng_Only_Mode [order 2] : [SoC < 0.1]
    Sport_Mode -> CS_Mode [order 2] : [SportModeEnabled == 0&&...
        | iceSystemStatus&&eSystemStatus]
    CS_Mode -> Sport_Mode [order 1] : [SportModeEnabled == 1&&...
        | iceSystemStatus&&eSystemStatus]
    CD_Mode -> VehReady.Clutch_Engage [order 1] : [(SW_CS_ON&&iceSystemStatus && ...
        | eSystemStatus)||...
        | SoC <CS_SOC_MIN&&iceSystemStatus == 2 && ...
        | eSystemStatus == 2]
    CS_Mode -> CD_Mode [order 3] : [(!SW_CS_ON&&SoC > CD_SOC_MIN&&...
        | eSystemStatus == 2) || ...
        | iceSystemStatus == 0]
    VehReady.Clutch_Engage -> CS_Mode : after(1,sec)
        | [ClutchEngage==0&&...
        | EngRunAtv == 1]
  VehOffOrAcc -> EnablePropulsion [order 3] : [KeyPos==3&&BrkPdlPos>10&&ShftLvrPos==1&&(~eSystemStatus&&iceSystemStatus)]
  (default) -> VehOffOrAcc
  VehOffOrAcc -> VehOn [order 2] : [KeyPos>= 1&&(eSystemStatus||iceSystemStatus)]
  Close_Contactors -> VehOffOrAcc [order 3] : [KeyPos < 1]
  VehOffOrAcc -> Charging [order 1] : [plugged]
  Charging -> VehOffOrAcc [order 2] : [plugged==0&&...
      | KeyPos==0]
  VehOn -> Close_Contactors : [INV_State==3]
  VehShutdown -> VehOffOrAcc [order 2] : after(1,sec)[plugged==0]
  Charging -> Close_Contactors [order 1] : [plugged==0&&...
      | KeyPos==1]
  Close_Contactors -> Charging [order 2] : [plugged]
  Close_Contactors -> EnablePropulsion [order 1] : [KeyPos==3&&BrkPdlPos>10&&...
      | ShftLvrPos==1]
  EnablePropulsion -> Charging [order 2] : [plugged]
  VehShutdown -> Charging [order 1] : [plugged]
  EnablePropulsion -> VehReady [order 1] : after(0.5,sec)
  VehReady -> Charging [order 1] : [plugged]
  VehReady -> VehShutdown [order 2] : [KeyPos < 2&&ShftLvrPos==1||...
      | (eSystemStatus==0&&iceSystemStatus==0)]
  data: APP function_input; EngSpeed function_input; T function_output; Shifter function_input; DrvIntdAxleTrq function_input; TransRatio function_input; T function_input; APP function_output; TransRatio function_input; EngSpeed function_input; EngApp function_output; MotorSpeed function_input; APP function_input; MotTrq function_output; ShftLvrPos function_input; DrvIntdAxleTrq function_input; TransRatio function_input; T function_output; BPP function_input; VehSpd function_input; ShftLvrPos function_input; MotSpeed function_input; TransRatio function_input; IntdAxleTrq function_input; T function_output; ShftLvrPos function_input; TransRatio function_input; T function_output; BPP function_input; VehSpd function_input; ShftLvrPos function_input; MotSpeed function_input; IntdAxleTrq function_input; TransRatio function_input; T function_output; APP function_input; Shifter function_input; MotSpeed function_input; DrvIntdAxleTrq function_input; TransRatio function_input; APP function_input; EngSpeed function_input; T function_output; Shifter function_input; DrvIntdAxleTrq function_input; TransRatio function_input; Trq function_input; APP function_output; TransRatio function_input; temp local double; EngSpeed function_input; EngApp function_output; MotorSpeed function_input; EngSpeed function_input; EngApp function_output; MotorSpeed function_input; Trq function_input; APP function_output; TransRatio function_input; Trq function_output; EngSpeed function_input; APP function_input; VehSpd function_input; ShftLvrPos function_input; DrvIntdAxleTrq function_input; TransRatio function_input; SOC function_input; APP function_input; MotTrq function_output; ShftLvrPos function_input; DrvIntdAxleTrq function_input; TransRatio function_input; SoC function_input; CS_On function_input; Faked_SoC function_input; MotSpd function_input; Trq function_input; T function_output; BPP function_input; VehSpd function_input; ShftLvrPos function_input; MotSpeed function_input; TransRatio function_input; IntdAxleTrq function_input; T function_output; ShftLvrPos function_input; TransRatio function_input; MotTrq function_output; APP function_input; DrvIntdAxleTrq function_input; TransRatio function_input; ShftLvrPos function_input; T function_output; BPP function_input; VehSpd function_input; ShftLvrPos function_input; MotSpeed function_input; TransRatio function_input; IntdAxleTrq function_input; T function_output; ShftLvrPos function_input; TransRatio function_input; EngSpeed function_input; EngApp function_output; MotorSpeed function_input; Trq function_input double size=1; APP function_output double size=1; TransRatio function_input double size=1; APP function_input double size=1; EngFdbkTrq function_input double size=1; MotTrq function_output double size=1; ShftLvrPos function_input double size=1; DrvIntdAxleTrq function_input double size=1; TransRatio function_input double size=1; Trq function_input double size=1; Trq function_output double size=1; EngSpeed function_input double size=1; APP function_input double size=1; VehSpd function_input double size=1; ShftLvrPos function_input double size=1; DrvIntdAxleTrq function_input double size=1; TransRatio function_input double size=1; T function_output double size=1; BPP function_input double size=1; VehSpd function_input double size=1; ShftLvrPos function_input double size=1; MotSpeed function_input double size=1; TransRatio function_input double size=1; IntdAxleTrq function_input double size=1; T function_output double size=1; ShftLvrPos function_input double size=1; TransRatio function_input double size=1; data local double; SportModeEnabled input boolean; TransEstGear input int8; mode output int8; powerMode output int8; closeMaincReq output double; EnablePrplsn output boolean; KeyPos input int8; BrkPdlPos input double; drvAPP input double; VehicleSpeed input double; EngSpd input double; MotSpd input double; ShftLvrPos input int8; EngAppReq output double; EngOnReq output boolean; MotTrqReq output double; EnableInverter output boolean; InverterEnabled input double; plugged input double; CD_SOC_MIN input double; CS_SOC_MIN input double; CS_SOC_MAX input double; EngRunAtv input boolean; SoC input double; EngTrq output double; DrvIntdAxleTrq input double; IntdAxleTrq input double; Faked_SoC input double; TransRatio input double; HV_Req output double; SW_CS_ON input boolean; SW_Engine_ON input boolean; RegenBrkDisable input boolean; Chg output double; Brkmode output double; Drvmode output double; eSystemStatus input; iceSystemStatus input; Drv_Mode local double; ABSAtv input boolean; Regen_fault input boolean; EngFdbkTrq input double; EngCtlTmp input; ClutchEngage output double; INV_State input; HoodStatus input

== stateflow chart Milford/Camaro Plant Model/Transmission/Soft TCM/6L45 Logic ==
  settings: sampleTime=0.04
  state Torque_Converter_Control [parallel]
    du:
    du:[lockup_thrsh]=calc_lockup(Gear_D, drvAPP);
    du:[unlock_thrsh]=calc_unlock(Gear_D, drvAPP);
    settings: executionOrder=1
    state lockup_th = calc_lockup(Gear, APP) [function]
    note: Lever Position:
        | 1 P
        | 2 R
        | 3 N
        | 4 D
        |
        | 1 clutch lock-up
        | 0 clutch unlock
    state Lock
      en:
      LockupCmd = 1;
    state Unlock
      en:
      LockupCmd = 0;
    state unlock_th = calc_unlock(Gear,APP) [function]
    (default) -> Unlock
    Unlock -> Lock : [(Gear_D >= 4 || drvBPP > 0) && VehicleSpeed > 20]
    Lock -> Unlock : [VehicleSpeed < 20 || drvBPP == 0 && drvAPP > 5 && Gear_D <= 3]
  state Gearbox_Control [parallel]
    settings: executionOrder=2
    state Shifter_Actuator [parallel]
      settings: executionOrder=1
      state Shifter_D
        du:
        TransEstGear = Gear_D;
      state Shifter_R
        en:
        TransEstGear = 14;
      state Shifter_N
        en:
        TransEstGear = 13;
      state Shifter_P
        en:
        TransEstGear = 15;
      (default) -> Shifter_P
      Shifter_D -> Shifter_N : [ShftLvrPos <= 3]
      Shifter_N -> Shifter_R [order 2] : [ShftLvrPos <= 2]
      Shifter_R -> Shifter_P [order 2] : [ShftLvrPos <= 1]
      Shifter_N -> Shifter_D [order 1] : [ShftLvrPos >= 4]
      Shifter_R -> Shifter_N [order 1] : [ShftLvrPos >= 3]
      Shifter_P -> Shifter_R : [ShftLvrPos >= 2]
    state Shift_Schedule [parallel]
      settings: executionOrder=2
      state Gear_State_D [parallel]
        settings: executionOrder=1
        state Gear_4th
          entry:
          Gear_D = 4;
        state Gear_3rd
          entry:
          Gear_D = 3;
        state Gear_6th
          entry:
          Gear_D = 6;
        state Gear_7th
          entry:
          Gear_D = 7;
        state Gear_8th
          entry:
          Gear_D = 8;
        state Gear_1st
          entry:
          Gear_D = 1;
        state Gear_5th
          entry:
          Gear_D = 5;
        state Gear_2nd
          entry:
          Gear_D  = 2;
        (default) -> Gear_1st
        Gear_2nd -> Gear_3rd [order 1] : UP
        Gear_7th -> Gear_8th [order 1] : UP
        Gear_4th -> Gear_5th [order 1] : UP
        Gear_5th -> Gear_6th [order 1] : UP
        Gear_6th -> Gear_7th [order 1] : UP
        Gear_3rd -> Gear_4th [order 1] : UP
        Gear_1st -> Gear_2nd : UP
        Gear_3rd -> Gear_2nd [order 2] : DOWN
        Gear_4th -> Gear_3rd [order 2] : DOWN
        Gear_2nd -> Gear_1st [order 2] : DOWN
        Gear_5th -> Gear_4th [order 2] : DOWN
        Gear_6th -> Gear_5th [order 2] : DOWN
        Gear_7th -> Gear_6th [order 2] : DOWN
        Gear_8th -> Gear_7th : DOWN
      state Gear_Transient_D [parallel]
        du:[up_thrsh]=calc_up(Gear_D, drvAPP);
        du:[down_thrsh]=calc_down(Gear_D, drvAPP);
        settings: executionOrder=2
        state steady_state
        state upshifting
        state downshifting
        (default) -> steady_state
        steady_state -> upshifting [order 1] : [VehicleSpeed > up_thrsh && Gear_D < 8]
        steady_state -> downshifting [order 2] : [VehicleSpeed < down_thrsh && Gear_D > 1]
        downshifting -> steady_state [order 1] : after(0.1,sec)
            | [VehicleSpeed <= down_thrsh]
            | {Gear_State_D.DOWN;}
        downshifting -> steady_state [order 2] : [VehicleSpeed > down_thrsh]
        upshifting -> steady_state [order 1] : after(0.1,sec)
            | [VehicleSpeed >= up_thrsh]
            | {Gear_State_D.UP;}
        upshifting -> steady_state [order 2] : [VehicleSpeed < up_thrsh]
      state PlotShiftSchedule [function]
      state up_th = calc_up(Gear, APP) [function]
      state down_th = calc_down(Gear, APP) [function]
  data: Gear function_input; APP function_input; lockup_th function_output; Gear function_input; APP function_input; unlock_th function_output; Gear function_input; APP function_input; up_th function_output; Gear function_input; APP function_input; down_th function_output; tc_lockup_thrsh input double; Gear_D local int8 =1; drvAPP input double [0..100]; VehicleSpeed input double; TransEstGear output int8; down_thrsh local double =0; up_thrsh local double =0; LockupCmd output boolean; tc_spd_in input double; tc_spd_out input double; drvBPP input double; ShftLvrPos input int8; lockup_thrsh local double; unlock_thrsh local double
  events: DOWN local EITHER_EDGE_EVENT; UP local EITHER_EDGE_EVENT

== stateflow chart Milford/Controller_with_Transmission_Manager1/HSC/Camaro Fault Detection/Component Diagnostic/Transmission Component Diagnostic/TCM_CompDia ==
  state TCM_Offline
    en: TCM_Status=0;
  state TCM_Limited [commented out]
    en: TCM_Status=1;
  state TCM_Online
    en: TCM_Status=2;
  (default) -> TCM_Offline
  TCM_Online -> TCM_Offline : [~TCMRollingAliveActive_SigValid||...
      | ~LvrPosTrnsShft_SigValid||...
      | ~TransEstGear_SigValid||...
      | ~LockupCmd_SigValid||VehDirFault]
  TCM_Offline -> TCM_Online : [TCMRollingAliveActive_SigValid&&...
      | LvrPosTrnsShft_SigValid&&TransEstGear_SigValid&&...
      | LockupCmd_SigValid&&VehDirFault==0]
  TCM_Limited -> TCM_Online [commented out]
  TCM_Online -> TCM_Limited [commented out]
  data: TCM_Status output; TCMRollingAliveActive_SigValid input; LvrPosTrnsShft_SigValid input; TransEstGear_SigValid input; LockupCmd_SigValid input; VehDirFault input

== stateflow chart Milford/Controller_with_Transmission_Manager1/HSC/Camaro Fault Detection/Input Conversions/TCM_Conversions/TCM_RollinAliveCounter/Rolling Alive Counter1 ==
  state RollingAliveCounter
    state Count1
      en: RollingAliveCnt=0;
    state Count2
      en: RollingAliveCnt=1;
    state Count3
      en: RollingAliveCnt=2;
    state Count4
      en: RollingAliveCnt=3;
    (default) -> Count1
    Count4 -> Count1 : after(0.01,sec)
    Count1 -> Count2 : after(0.01,sec)
    Count2 -> Count3 : after(0.01,sec)
    Count3 -> Count4 : after(0.01,sec)
  data: RollingAliveCnt output double

== stateflow chart Milford/Controller_with_Transmission_Manager1/HSC/Camaro Fault Detection/Signal Diagnostic/Engine Signal Diagnostic/Engine_Temp[DegC] ==
  state AboveMax
    en: EngTempRange=3;
  state HighRange
    en: EngTempRange=2;
  state NormalRange
    en: EngTempRange=1;
  HighRange -> AboveMax [order 2] : [Engine_Temp_DegC>120]
  AboveMax -> HighRange : [Engine_Temp_DegC<120]
  NormalRange -> HighRange [order 1] : [Engine_Temp_DegC>100&&Engine_Temp_DegC<120]
  HighRange -> NormalRange [order 1] : [Engine_Temp_DegC<=100]
  NormalRange -> NormalRange [order 2] : [clearFaults==1]
      | {EngTempRange=1;}
  (default) -> NormalRange
  data: clearFaults input; Engine_Temp_DegC input; EngTempRange output; data local
